simulink model "VSI_v_loop_tfvdqvdqref_delay"  (Simulink 7.6)
settings: Solver=ode23t  StartTime=0.0  StopTime=0.5  MaxStep=25e-6  RelTol=1e-4  AbsTol=1e-5
values from neighbouring files (symbols this model uses):
  C = 21.308e-6    (= 2.1308e-05)    [Current_Loop_Design.m]    (also in VSI_Controller_Design.m = 3.13e-05; VSI_TFs_i_loop.m = 2.2e-05; VSI_TFs_o_loop.m = 4.13e-05; VSI_TFs_v_loop.m = 4.1308e-05)
  kii = 2*pi*800*(RL)/Vdc*10    (= 27.9252680319)    [Current_Loop_Design.m]    (also in VSI_TFs_o_loop.m; ZVSI_il_tf_cal_sim_comp_frd_model_v1.m = 0.173333333333; ZVSI_ol_tf_cal_sim_comp_frd_model_v1.m = 0.00279252680319; ZVSI_vil_tf_cal_frd_model_Monte_Carlo.m = 93.6)
  kiv = 130    [ZVSI_il_tf_cal_sim_comp_frd_model_v1.m]    (also in ZVSI_ol_tf_cal_sim_comp_frd_model_v1.m = 83.7758040957; ZVSI_vil_tf_cal_frd_model_Monte_Carlo.m = 75.3982236862; ZVSI_vil_tf_cal_sim_comp_frd_model_v1.m = 130.8996939; ZVSI_vil_tf_cal_sim_comp_frd_model_v2.m = 2*pi*fv/R)
  kpi = 2*pi*800*L/Vdc*0.5    (= 0.010239264945)    [Current_Loop_Design.m]    (also in VSI_TFs_o_loop.m; ZVSI_il_tf_cal_sim_comp_frd_model_v1.m = 1.43866666667e-05; ZVSI_ol_tf_cal_sim_comp_frd_model_v1.m = 0.0093084226773; ZVSI_vil_tf_cal_frd_model_Monte_Carlo.m = 0.0077688)
  kpv = 130*2.2e-5    (= 0.00286)    [ZVSI_il_tf_cal_sim_comp_frd_model_v1.m]    (also in ZVSI_ol_tf_cal_sim_comp_frd_model_v1.m = 0.013110913341; ZVSI_vil_tf_cal_frd_model_Monte_Carlo.m = 0.0338443776571; ZVSI_vil_tf_cal_sim_comp_frd_model_v1.m = 0.049480084294; ZVSI_vil_tf_cal_sim_comp_frd_model_v2.m = 2*pi*fv*C)
  L = (0.75879e-3)/(2/3)    (= 0.001138185)    [Current_Loop_Design.m]    (also in VSI_Controller_Design.m = 0.0011; VSI_TFs_i_loop.m = 0.0012; VSI_TFs_o_loop.m = 0.0011; VSI_TFs_v_loop.m = 0.0011)
  R = 15    [Current_Loop_Design.m]    (also in ZVSI_il_tf_cal_sim_comp_frd_model_v1.m; ZVSI_ol_tf_cal_sim_comp_frd_model_v1.m; ZVSI_vil_tf_cal_frd_model_Monte_Carlo.m = R_rec(i); ZVSI_vil_tf_cal_sim_comp_frd_model_v1.m = 12)
  RL = 80e-3    (= 0.08)    [Current_Loop_Design.m]    (also in ZVSI_il_tf_cal_sim_comp_frd_model_v1.m = 0.15; ZVSI_ol_tf_cal_sim_comp_frd_model_v1.m = 1.5e-05; ZVSI_vil_tf_cal_frd_model_Monte_Carlo.m = 0.13; ZVSI_vil_tf_cal_sim_comp_frd_model_v1.m = 0.13)
  Tdelay = 1.5*Tsw    (= 7.5e-05)    [Current_Loop_Design.m]    (also in VSI_Controller_Design.m = 2.5e-05; VSI_TFs_i_loop.m = 5e-05; VSI_TFs_o_loop.m; VSI_TFs_v_loop.m = 5e-05)
  Tdelay1 = 0.6*Tsw    (= 3e-05)    [vsi_conv_init.m]
  Vdc = 270    [Current_Loop_Design.m]    (also in VSI_Controller_Design.m; VSI_TFs_i_loop.m; VSI_TFs_o_loop.m; VSI_TFs_v_loop.m)
  Vdcref = 270    [Current_Loop_Design.m]    (also in ZVSI_il_tf_cal_sim_comp_frd_model_v1.m; ZVSI_ol_tf_cal_sim_comp_frd_model_v1.m; ZVSI_vil_tf_cal_frd_model_Monte_Carlo.m; ZVSI_vil_tf_cal_sim_comp_frd_model_v1.m)
  Vdref = Vsdq(1)    [Current_Loop_Design.m]    (also in ZVSI_il_tf_cal_sim_comp_frd_model_v1.m; ZVSI_ol_tf_cal_sim_comp_frd_model_v1.m; ZVSI_vil_tf_cal_frd_model_Monte_Carlo.m; ZVSI_vil_tf_cal_sim_comp_frd_model_v1.m)
  Vqref = Vsdq(2)    [Current_Loop_Design.m]    (also in ZVSI_il_tf_cal_sim_comp_frd_model_v1.m; ZVSI_ol_tf_cal_sim_comp_frd_model_v1.m; ZVSI_vil_tf_cal_frd_model_Monte_Carlo.m; ZVSI_vil_tf_cal_sim_comp_frd_model_v1.m)
  w = 2*pi*fline    (= 2513.27412287)    [Current_Loop_Design.m]    (also in ZVSI_il_tf_cal_sim_comp_frd_model_v1.m = 15791.3670417; ZVSI_ol_tf_cal_sim_comp_frd_model_v1.m = 15791.3670417; ZVSI_vil_tf_cal_frd_model_Monte_Carlo.m = 15791.3670417; ZVSI_vil_tf_cal_sim_comp_frd_model_v1.m = 15791.3670417)
libraries: powerlib x22
settings Model: Creator=marko  LastModifiedBy=wenbo  BufferReuse=off
settings OptimizationCC: BlockReduction=off  InlineParams=on  BufferReuse=off
settings DebuggingCC: AlgebraicLoopMsg=none  SolverPrmCheckMsg=none  UnconnectedInputMsg=none  UnconnectedOutputMsg=none  UnconnectedLineMsg=none  StrictBusMsg=Warning

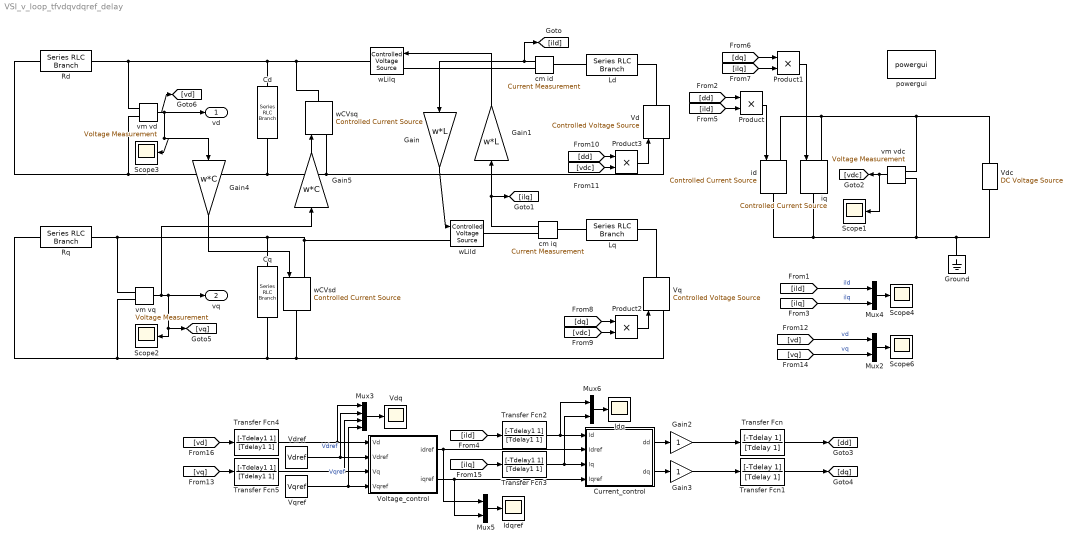
== system VSI_v_loop_tfvdqvdqref_delay ==
  Cd : powerlib/Elements/Series RLC Branch  DialogController=POWERSYS.PowerSysDialog  PhysicalDomain=powersysdomain  SubClassName=unknown  LeftPortType=p1  RightPortType=p1  LConnTagsString=__new0  RConnTagsString=__new0  BranchType=C  Resistance=1  Inductance=1e-3  SetiL0=off  InitialCurrent=0  Capacitance=C  Setx0=off  InitialVoltage=0  Measurements=None
  Cq : powerlib/Elements/Series RLC Branch  DialogController=POWERSYS.PowerSysDialog  PhysicalDomain=powersysdomain  SubClassName=unknown  LeftPortType=p1  RightPortType=p1  LConnTagsString=__new0  RConnTagsString=__new0  BranchType=C  Resistance=1  Inductance=1e-3  SetiL0=off  InitialCurrent=0  Capacitance=C  Setx0=off  InitialVoltage=0  Measurements=None
  Current_control : Subsystem
  Gain : Gain  Gain=w*L
  Gain1 : Gain  Gain=w*L
  Gain2 : Gain
  Gain3 : Gain
  Gain4 : Gain  Gain=w*C
  Gain5 : Gain  Gain=w*C
  Ground : powerlib/Elements/Ground  DialogController=POWERSYS.PowerSysDialog  PhysicalDomain=powersysdomain  SubClassName=unknown  LeftPortType=p1  RightPortType=p1  LConnTagsString=a
  Idq : Scope
      settings: YMin=5.5  YMax=6.65  SaveName=ildq_matlab5  DataFormat=Array
  Idqref : Scope
      settings: YMin=4.4  YMax=5.35  SaveName=ildq_matlab4  DataFormat=Array
  Ld : powerlib/Elements/Series RLC Branch  DialogController=POWERSYS.PowerSysDialog  PhysicalDomain=powersysdomain  SubClassName=unknown  LeftPortType=p1  RightPortType=p1  LConnTagsString=__new0  RConnTagsString=__new0  BranchType=RL  Resistance=RL  Inductance=L  SetiL0=off  InitialCurrent=0  Capacitance=1e-6  Setx0=off  InitialVoltage=0  Measurements=None
  Lq : powerlib/Elements/Series RLC Branch  DialogController=POWERSYS.PowerSysDialog  PhysicalDomain=powersysdomain  SubClassName=unknown  LeftPortType=p1  RightPortType=p1  LConnTagsString=__new0  RConnTagsString=__new0  BranchType=RL  Resistance=RL  Inductance=L  SetiL0=off  InitialCurrent=0  Capacitance=1e-6  Setx0=off  InitialVoltage=0  Measurements=None
  Mux{2,4..6} (4 alike) : Mux  Inputs=2
  Mux3 : Mux
  Product{,1..3} (4 alike) : Product  RndMeth=Zero
  Rd : powerlib/Elements/Series RLC Branch  DialogController=POWERSYS.PowerSysDialog  PhysicalDomain=powersysdomain  SubClassName=unknown  LeftPortType=p1  RightPortType=p1  LConnTagsString=__new0  RConnTagsString=__new0  BranchType=R  Resistance=R  Inductance=1e-3  SetiL0=off  InitialCurrent=0  Capacitance=1e-6  Setx0=off  InitialVoltage=0  Measurements=None
  Rq : powerlib/Elements/Series RLC Branch  DialogController=POWERSYS.PowerSysDialog  PhysicalDomain=powersysdomain  SubClassName=unknown  LeftPortType=p1  RightPortType=p1  LConnTagsString=__new0  RConnTagsString=__new0  BranchType=R  Resistance=R  Inductance=1e-3  SetiL0=off  InitialCurrent=0  Capacitance=1e-6  Setx0=off  InitialVoltage=0  Measurements=None
  Scope{1..4,6} (5 alike) : Scope
      Scope1 settings: YMin=270  YMax=270  SaveName=ildq_matlab  DataFormat=Array
      Scope2 settings: YMin=256.5  YMax=283.5  SaveName=ildq_matlab1  DataFormat=Array
      Scope3 settings: YMin=256.5  YMax=283.5  SaveName=ildq_matlab2  DataFormat=Array
      Scope4 settings: YMin=-0.25  YMax=5.25  SaveName=ildq_matlab3  DataFormat=Array
      Scope6 settings: YMin=0  YMax=100  SaveName=ildq_matlab8  DataFormat=Array
  Transfer Fcn : TransferFcn  Numerator=[-Tdelay 1]  Denominator=[Tdelay 1]
  Transfer Fcn1 : TransferFcn  Numerator=[-Tdelay 1]  Denominator=[Tdelay 1]
  Transfer Fcn{2..5} (4 alike) : TransferFcn  Numerator=[-Tdelay1 1]  Denominator=[Tdelay1 1]
  Vd : powerlib/Electrical Sources/Controlled Voltage Source  DialogController=POWERSYS.PowerSysDialog  SystemSampleTime=-1  Initialize=on  Source_Type=DC  Amplitude=0  Phase=0  Frequency=0  Measurements=None
  Vdc : powerlib/Electrical Sources/DC Voltage Source  DialogController=POWERSYS.PowerSysDialog  SystemSampleTime=-1  Amplitude=Vdc  Measurements=None
  Vdq : Scope
      settings: YMin=-20  YMax=110  SaveName=ildq_matlab6  DataFormat=Array
  Vdref : Constant  Value=Vdref
  Voltage_control : Subsystem
  Vq : powerlib/Electrical Sources/Controlled Voltage Source  DialogController=POWERSYS.PowerSysDialog  SystemSampleTime=-1  Initialize=on  Source_Type=DC  Amplitude=0  Phase=0  Frequency=0  Measurements=None
  Vqref : Constant  Value=Vqref
  cm id : powerlib/Measurements/Current Measurement  DialogController=POWERSYS.PowerSysDialog  SystemSampleTime=-1  PhasorSimulation=off  OutputType=Complex  PSBequivalent=0
  cm iq : powerlib/Measurements/Current Measurement  DialogController=POWERSYS.PowerSysDialog  SystemSampleTime=-1  PhasorSimulation=off  OutputType=Complex  PSBequivalent=0
  id : powerlib/Electrical Sources/Controlled Current Source  DialogController=POWERSYS.PowerSysDialog  SystemSampleTime=-1  Initialize=on  Source_Type=DC  Amplitude=0  Phase=0  Frequency=0  Measurements=None
  iq : powerlib/Electrical Sources/Controlled Current Source  DialogController=POWERSYS.PowerSysDialog  SystemSampleTime=-1  Initialize=on  Source_Type=DC  Amplitude=0  Phase=0  Frequency=0  Measurements=None
  powergui : powerlib/powergui  Priority=1  SystemSampleTime=-1  SimulationMode=Continuous  SampleTime=50e-6  frequency=60  SPID=off  DisableSnubberDevices=off  DisableRonSwitches=off  DisableVfSwitches=off  SwTol=0  Interpol=off  frequencyindice=0  echomessages=off  HookPort=off  DisplayEquations=off  FunctionMessages=off  EnableUseOfTLC=off  x0status=blocks  RestoreLinks=warning  ResistiveCurrentMeasurement=off  Frange=[0:2:500]  Ylog=off  Xlog=on  ShowGrid=off  save=off  variable=ZData  ZoomFFT=on  StartTime=0.0  cycles=1  DisplayStyle=1  fundamental=60  FreqAxis=off  MaxFrequency=1000  frequencyindicesteady=1  RmsSteady=1  display=off  Ts=0  methode=off
  vm vd : powerlib/Measurements/Voltage Measurement  DialogController=POWERSYS.PowerSysDialog  SystemSampleTime=-1  PhasorSimulation=off  OutputType=Complex  PSBequivalent=0
  vm vdc : powerlib/Measurements/Voltage Measurement  DialogController=POWERSYS.PowerSysDialog  SystemSampleTime=-1  PhasorSimulation=off  OutputType=Complex  PSBequivalent=0
  vm vq : powerlib/Measurements/Voltage Measurement  DialogController=POWERSYS.PowerSysDialog  SystemSampleTime=-1  PhasorSimulation=off  OutputType=Complex  PSBequivalent=0
  wCVsd : powerlib/Electrical Sources/Controlled Current Source  DialogController=POWERSYS.PowerSysDialog  SystemSampleTime=-1  Initialize=on  Source_Type=DC  Amplitude=0  Phase=0  Frequency=0  Measurements=None
  wCVsq : powerlib/Electrical Sources/Controlled Current Source  DialogController=POWERSYS.PowerSysDialog  SystemSampleTime=-1  Initialize=on  Source_Type=DC  Amplitude=0  Phase=0  Frequency=0  Measurements=None
  wLild : powerlib/Electrical Sources/Controlled Voltage Source  DialogController=POWERSYS.PowerSysDialog  SystemSampleTime=-1  Initialize=on  Source_Type=DC  Amplitude=0  Phase=0  Frequency=0  Measurements=None
  wLilq : powerlib/Electrical Sources/Controlled Voltage Source  DialogController=POWERSYS.PowerSysDialog  SystemSampleTime=-1  Initialize=on  Source_Type=DC  Amplitude=0  Phase=0  Frequency=0  Measurements=None
  vd : Outport
  vq : Outport  Port=2
  wires:
  Product/1 -> id/1
  [dd] -> Product/1
  [ild] -> Product/2
  Product1/1 -> iq/1
  [dq] -> Product1/1
  [ilq] -> Product1/2
  [dq] -> Product2/1
  [vdc] -> Product2/2
  Product2/1 -> Vq/1
  [dd] -> Product3/1
  [vdc] -> Product3/2
  Product3/1 -> Vd/1
  vm vd/1 -> vd/1, [vd], Gain4/1, Scope3/1
  vm vq/1 -> Gain5/1, vq/1, [vq], Scope2/1
  vm vdc/1 -> [vdc], Scope1/1
  cm iq/1 -> Gain1/1, [ilq]
  Gain1/1 -> wLilq/1
  cm id/1 -> Gain/1, [ild]
  Gain/1 -> wLild/1
  Gain4/1 -> wCVsd/1
  Gain5/1 -> wCVsq/1
  [ild] -> Mux4/1  "ild"
  [ilq] -> Mux4/2  "ilq"
  Mux4/1 -> Scope4/1
  [vd] -> Mux2/1  "vd"
  [vq] -> Mux2/2  "vq"
  Mux2/1 -> Scope6/1
  [ild] -> Transfer Fcn2/1
  [ilq] -> Transfer Fcn3/1
  Current_control/1(dd) -> Gain2/1
  Current_control/2(dq) -> Gain3/1
  Voltage_control/2(iqref) -> Current_control/4(Iqref), Mux5/2
  Mux6/1 -> Idq/1
  Gain2/1 -> Transfer Fcn/1
  Gain3/1 -> Transfer Fcn1/1
  Vqref/1 -> Voltage_control/4(Vqref), Mux3/4  "Vqref"
  Vdref/1 -> Voltage_control/2(Vdref), Mux3/2  "Vdref"
  [vd] -> Transfer Fcn4/1
  [vq] -> Transfer Fcn5/1
  Voltage_control/1(idref) -> Current_control/2(Idref), Mux5/1
  Mux3/1 -> Vdq/1
  Mux5/1 -> Idqref/1
  Transfer Fcn/1 -> [dd]
  Transfer Fcn1/1 -> [dq]
  Transfer Fcn2/1 -> Mux6/1, Current_control/1(Id)
  Transfer Fcn3/1 -> Mux6/2, Current_control/3(Iq)
  Transfer Fcn4/1 -> Voltage_control/1(Vd), Mux3/1
  Transfer Fcn5/1 -> Voltage_control/3(Vq), Mux3/3
  connections:
  Vq/LConn1 -- wCVsd/RConn1 -- Cq/RConn1 -- Rq/LConn1 -- vm vq/LConn2
  iq/RConn1 -- id/RConn1 -- vm vdc/LConn2 -- Ground/LConn1 -- Vdc/LConn1
  Cq/LConn1 -- wCVsd/LConn1 -- wLild/LConn1 -- Rq/RConn1 -- vm vq/LConn1
  wLilq/LConn1 -- cm id/RConn1
  wLild/RConn1 -- cm iq/RConn1
  cm iq/LConn1 -- Lq/LConn1
  cm id/LConn1 -- Ld/LConn1
  Ld/RConn1 -- Vd/RConn1
  Lq/RConn1 -- Vq/RConn1
  Vdc/RConn1 -- iq/LConn1 -- id/LConn1 -- vm vdc/LConn1
  Rd/RConn1 -- wCVsq/RConn1 -- wLilq/RConn1 -- Cd/LConn1 -- vm vd/LConn1
  Vd/LConn1 -- wCVsq/LConn1 -- Cd/RConn1 -- vm vd/LConn2 -- Rd/LConn1

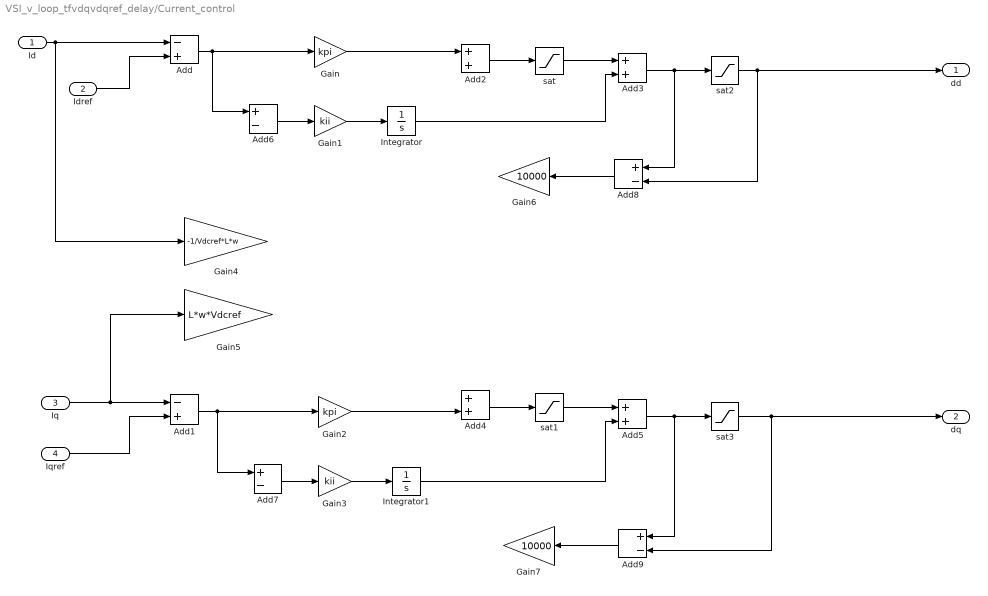
== system VSI_v_loop_tfvdqvdqref_delay/Current_control ==
  Id : Inport
  Idref : Inport  Port=2
  Iq : Inport  Port=3
  Iqref : Inport  Port=4
  Add : Sum  Inputs=-+
  Add1 : Sum  Inputs=-+
  Add{2..5} (4 alike) : Sum
  Add{6..9} (4 alike) : Sum  Inputs=+-
  Gain : Gain  Gain=kpi
  Gain1 : Gain  Gain=kii
  Gain2 : Gain  Gain=kpi
  Gain3 : Gain  Gain=kii
  Gain4 : Gain  Gain=-1/Vdcref*L*w
  Gain5 : Gain  Gain=L*w*Vdcref
  Gain6 : Gain  Gain=10000
  Gain7 : Gain  Gain=10000
  Integrator : Integrator
  Integrator1 : Integrator
  sat{,1..3} (4 alike) : Saturate  UpperLimit=1  LowerLimit=-1
  dd : Outport
  dq : Outport  Port=2
  wires:
  Id/1 -> Gain4/1, Add/1
  Idref/1 -> Add/2
  Iq/1 -> Gain5/1, Add1/1
  Iqref/1 -> Add1/2
  Add/1 -> Gain/1, Add6/1
  Gain1/1 -> Integrator/1
  Add2/1 -> sat/1
  sat/1 -> Add3/1
  Integrator/1 -> Add3/2
  Gain/1 -> Add2/1
  Add1/1 -> Gain2/1, Add7/1
  Gain3/1 -> Integrator1/1
  Gain2/1 -> Add4/2
  Add4/1 -> sat1/1
  sat1/1 -> Add5/1
  Integrator1/1 -> Add5/2
  sat2/1 -> Add8/2, dd/1
  Add5/1 -> sat3/1, Add9/1
  sat3/1 -> Add9/2, dq/1
  Add6/1 -> Gain1/1
  Add7/1 -> Gain3/1
  Add3/1 -> Add8/1, sat2/1
  Add8/1 -> Gain6/1
  Add9/1 -> Gain7/1

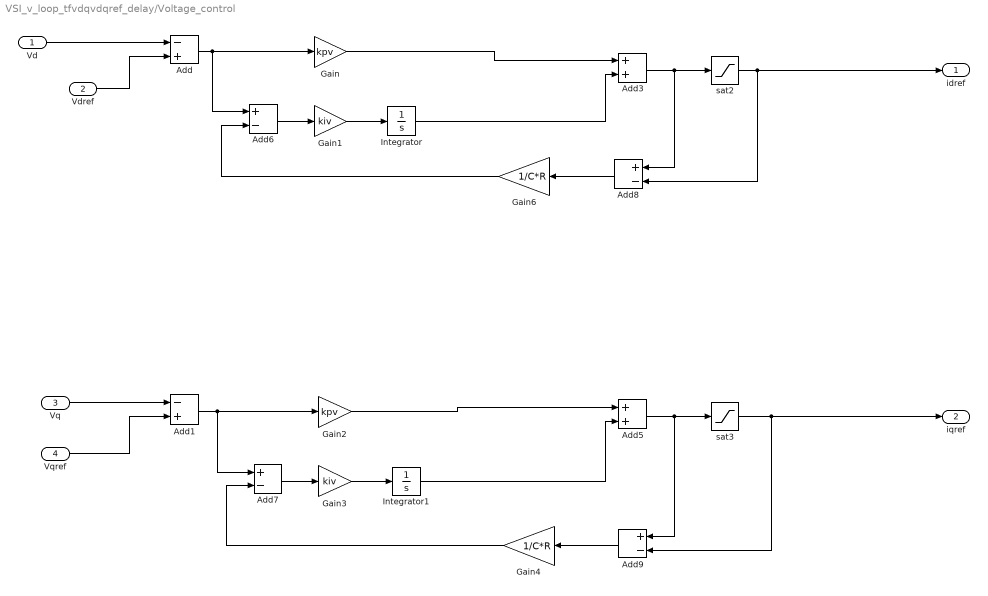
== system VSI_v_loop_tfvdqvdqref_delay/Voltage_control ==
  Vd : Inport
  Vdref : Inport  Port=2
  Vq : Inport  Port=3
  Vqref : Inport  Port=4
  Add : Sum  Inputs=-+
  Add1 : Sum  Inputs=-+
  Add3 : Sum
  Add5 : Sum
  Add{6..9} (4 alike) : Sum  Inputs=+-
  Gain : Gain  Gain=kpv
  Gain1 : Gain  Gain=kiv
  Gain2 : Gain  Gain=kpv
  Gain3 : Gain  Gain=kiv
  Gain4 : Gain  Gain=1/C*R
  Gain6 : Gain  Gain=1/C*R
  Integrator : Integrator
  Integrator1 : Integrator
  sat2 : Saturate  UpperLimit=40  LowerLimit=-40
  sat3 : Saturate  UpperLimit=40  LowerLimit=-40
  idref : Outport
  iqref : Outport  Port=2
  wires:
  Gain4/1 -> Add7/2
  Gain6/1 -> Add6/2
  Add9/1 -> Gain4/1
  Add8/1 -> Gain6/1
  Add3/1 -> sat2/1, Add8/1
  Add7/1 -> Gain3/1
  Add6/1 -> Gain1/1
  sat3/1 -> iqref/1, Add9/2
  Add5/1 -> Add9/1, sat3/1
  sat2/1 -> idref/1, Add8/2
  Integrator1/1 -> Add5/2
  Gain2/1 -> Add5/1
  Gain3/1 -> Integrator1/1
  Add1/1 -> Add7/1, Gain2/1
  Gain/1 -> Add3/1
  Integrator/1 -> Add3/2
  Gain1/1 -> Integrator/1
  Add/1 -> Add6/1, Gain/1
  Vqref/1 -> Add1/2
  Vq/1 -> Add1/1
  Vdref/1 -> Add/2
  Vd/1 -> Add/1
